simulink model "passivityBasedControl"  (Simulink 8.3)
settings: Solver=ode45  StartTime=0.0  StopTime=100  RelTol=1e-3
values from neighbouring files (symbols this model uses):
  jointModel = B12_rigid_gearbox    [configPassivityBasedController.m]
  KB = jointModel.k_b    [configPassivityBasedController.m]
  Kd = K(3)    [configPassivityBasedController.m]
  Kp = K(1)    [configPassivityBasedController.m]
  KS = K(4)    [configPassivityBasedController.m]
  KT = K(2)    [configPassivityBasedController.m]
undefined symbols (not defined in the file): my_joint
libraries: simulink x1, SEA_library_models x1, cstblocks x1
settings Model: Creator=joern  LastModifiedBy=joern
settings DataIOCC: SignalLoggingSaveFormat=Dataset
settings DebuggingCC: UnderspecifiedInitializationDetection=Simplified  MergeDetectMultiDrivingBlocksExec=error  FrameProcessingCompatibilityMsg=error  StateNameClashWarn=none
settings GRTTargetCC: CombineOutputUpdateFcns=on  GRTInterface=off
settings ConfigComp: CovMetricSettings=dw  CovHtmlReporting=on  CovSaveCumulativeToWorkspaceVar=on  CovSaveSingleToWorkspaceVar=on  CovModelRefEnable=Off  CovExternalEMLEnable=off

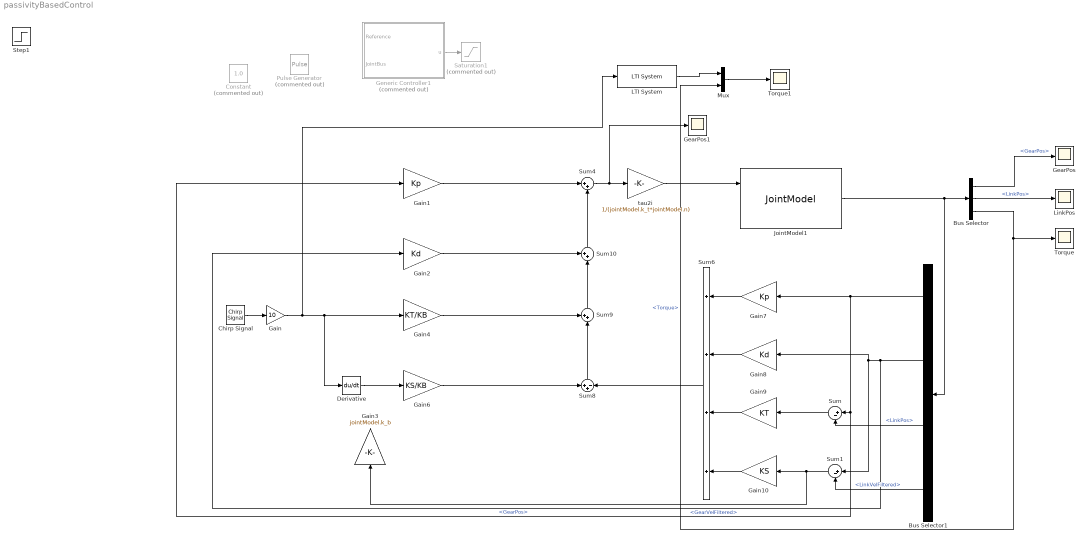
== system passivityBasedControl ==
  Bus Selector : BusSelector  OutputSignals=GearPos,LinkPos,Torque
  Bus Selector1 : BusSelector  OutputSignals=GearPos,GearVelFiltered,LinkPos,LinkVelFiltered
  Chirp Signal : simulink/Sources/Chirp Signal  f1=0.1  T=100  f2=100
  Constant : Constant  Commented=on  Value=1.0
  Derivative : Derivative
  Gain : Gain  Gain=10  SampleTime=jointModel.Ts
  Gain1 : Gain  Gain=Kp
  Gain10 : Gain  Gain=KS
  Gain2 : Gain  Gain=Kd
  Gain3 : Gain  Gain=jointModel.k_b
  Gain4 : Gain  Gain=KT/KB
  Gain6 : Gain  Gain=KS/KB
  Gain7 : Gain  Gain=Kp
  Gain8 : Gain  Gain=Kd
  Gain9 : Gain  Gain=KT
  GearPos : Scope
      settings: YMin=0.0001025  YMax=0.0001095
  GearPos1 : Scope
      settings: YMin=-30  YMax=30
  Generic Controller1 : Subsystem  Commented=on  mask{jointObj=my_joint}
      mask prompts: jointObj "Joint Object"
      mask init:
      | % Get linear dynamics matrices
      | [A, B, C, I, D, K] = jointObj.getDynamicsMatrices();
  JointModel1 : SEA_library_models/Joint models/JointModel  jointObj=jointModel  fc_vel=100  fc_torque=100  input_delay=0  output_delay=0  input_noise_enabled=off  output_noise_enabled=off  var_u=0.12^2  var_y=1.8e-10
  LTI System : cstblocks/LTI System  sys=clsys  IC=[]
  LinkPos : Scope
  Mux : Mux  Inputs=2
  Pulse Generator : DiscretePulseGenerator  Commented=on  PulseType=Time based  Period=10  PulseWidth=0.1
  Saturation1 : Saturate  Commented=on  UpperLimit=40  LowerLimit=-40
  Step1 : Step
  Sum : Sum  Inputs=|+-
  Sum1 : Sum  Inputs=|+-
  Sum10 : Sum  Inputs=++|
  Sum4 : Sum  Inputs=|++
  Sum6 : Sum  Inputs=++++
  Sum8 : Sum  Inputs=++-
  Sum9 : Sum  Inputs=++|
  Torque : Scope
      settings: TimeRange=60  YMin=-2.25  YMax=2.25
  Torque1 : Scope
      settings: TimeRange=60  YMin=-3.25e+35  YMax=2.5e+34  SaveName=ScopeData2
  tau2i : Gain  Gain=1/(jointModel.k_t*jointModel.n)
  wires:
  JointModel1/1 -> Bus Selector1/1, Bus Selector/1
  Bus Selector/2 -> LinkPos/1  "<LinkPos>"
  Bus Selector/3 -> Mux/2, Torque/1  "<Torque>"
  Bus Selector/1 -> GearPos/1  "<GearPos>"
  Generic Controller1/1(u) -> Saturation1/1
  Chirp Signal/1 -> Gain/1
  Bus Selector1/1 -> Gain1/1, Sum/1, Gain7/1  "<GearPos>"
  Bus Selector1/2 -> Gain2/1, Sum1/1, Gain8/1  "<GearVelFiltered>"
  Bus Selector1/3 -> Sum/2  "<LinkPos>"
  Sum/1 -> Gain9/1
  Bus Selector1/4 -> Sum1/2  "<LinkVelFiltered>"
  Sum1/1 -> Gain3/1, Gain10/1
  Sum4/1 -> GearPos1/1, tau2i/1
  Gain7/1 -> Sum6/1
  Gain8/1 -> Sum6/2
  Gain9/1 -> Sum6/3
  Gain10/1 -> Sum6/4
  Gain6/1 -> Sum8/1
  Sum6/1 -> Sum8/3
  Sum8/1 -> Sum9/2
  Gain4/1 -> Sum9/1
  Gain2/1 -> Sum10/1
  Sum9/1 -> Sum10/2
  Sum10/1 -> Sum4/2
  Gain1/1 -> Sum4/1
  tau2i/1 -> JointModel1/1
  Gain/1 -> LTI System/1, Derivative/1, Gain4/1
  Derivative/1 -> Gain6/1
  LTI System/1 -> Mux/1
  Mux/1 -> Torque1/1

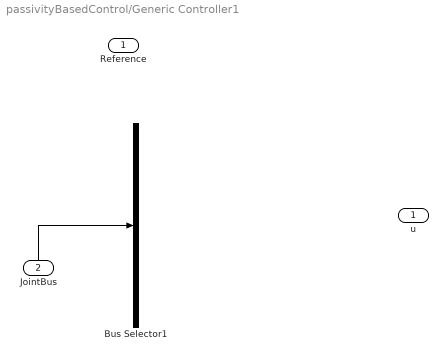
== system passivityBasedControl/Generic Controller1 ==
  Reference : Inport
  JointBus : Inport  Port=2
  Bus Selector1 : BusSelector  OutputSignals=GearPos,LinkPos,Torque
  u : Outport
  wires:
  JointBus/1 -> Bus Selector1/1

== matlab function JointModel1/nonLinDynamicsFcn ==
  data: x input double; tau output double
function tau = nonLinDynamics(x)
%#codegen

params.verbose = 0.000000;
params.debug = 0.000000;
params.a_CU = 0.003900;
params.c_CU = 380.000000;
params.c_FE = 460.000000;
params.isSym = 0.000000;
params.diam = 100.000000;
params.len = 150.000000;
params.m = 2.000000;
params.I_m = 0.550000;
params.I_g = 0.263000;
params.I_b = 1.000000;
params.k_g = 30000.000000;
params.k_b = 1623.000000;
params.d_m = 0.000000;
params.d_g = 2.515400;
params.d_b = 0.000000;
params.d_m_n = 0.000000;
params.d_g_n = 2.694000;
params.d_b_n = 0.000000;
params.d_mg = 0.000000;
params.d_gb = 0.000000;
params.d_cm = 0.000000;
params.d_cg = 0.816300;
params.d_cb = 0.000000;
params.d_cm_n = 0.000000;
params.d_cg_n = 0.889200;
params.d_cb_n = 0.000000;
params.d_s = 1.800000;
params.v_s = 0.010000;
params.cog_a1 = 1.500000;
params.cog_a2 = 0.000000;
params.cog_f = 1300.000000;
params.n = 100.000000;
params.k_t = 0.044500;
params.r = 0.088500;
params.x = 0.000140;
params.v_0 = 24.000000;
params.i_p = 40.000000;
params.dq_p = 5.860000;
params.r_th1 = 0.290000;
params.r_th2 = 3.450000;
params.T_thw = 3.960000;
params.T_thm = 1240.000000;
params.Tmp_WMax = 120.000000;
params.Tmp_ANom = 25.000000;
params.name = 'B12_rigid_gearbox';
params.paramName = 'B12';
params.modelName = 'rigid_gearbox';
params.nonlinearModelName = '';
params.Ts = 0.000500;
tau =zeros(size(x));
	end
